simulink model "motorCC"  (R2017b)
settings: Solver=VariableStepAuto  StartTime=0.0  StopTime=5.0  RelTol=1e-3
settings Model: Creator=Sofia  LastModifiedBy=Sofia

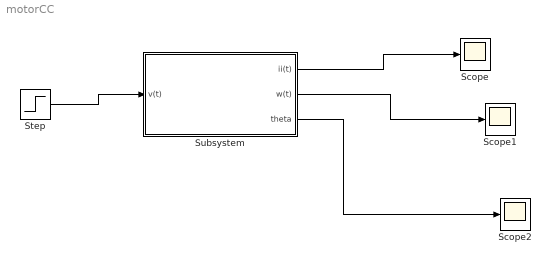
== system motorCC ==
  Scope : Scope
  Scope1 : Scope
  Scope2 : Scope
  Step : Step  After=5  SampleTime=0
  Subsystem : Subsystem
  wires:
  Step/1 -> Subsystem/1(v(t))
  Subsystem/1(ii(t)) -> Scope/1
  Subsystem/2(w(t)) -> Scope1/1
  Subsystem/3(theta) -> Scope2/1

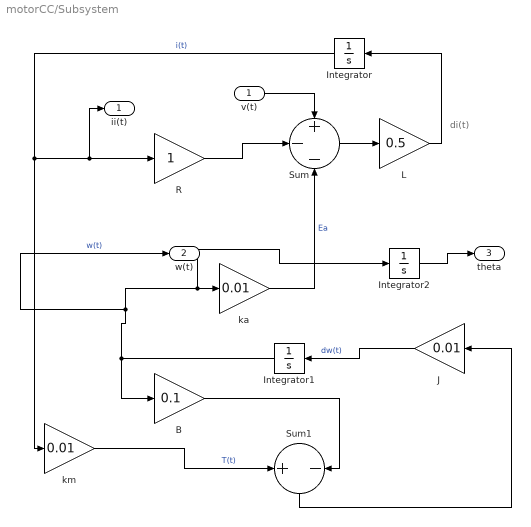
== system motorCC/Subsystem ==
  note: di(t)
  v(t) : Inport
  B : Gain  Gain=0.1
  Integrator : Integrator
  Integrator1 : Integrator
  Integrator2 : Integrator
  J : Gain  Gain=0.01
  L : Gain  Gain=0.5
  R : Gain
  Sum : Sum  Inputs=+--
  Sum1 : Sum  Inputs=+-
  ka : Gain  Gain=0.01
  km : Gain  Gain=0.01
  ii(t) : Outport
  w(t) : Outport  Port=2
  theta : Outport  Port=3
  wires:
  Integrator1/1 -> B/1, w(t)/1, Integrator2/1, ka/1  "w(t)"
  Integrator/1 -> km/1, ii(t)/1, R/1  "i(t)"
  Sum/1 -> L/1
  ka/1 -> Sum/3  "Ea"
  Integrator2/1 -> theta/1
  v(t)/1 -> Sum/1
  L/1 -> Integrator/1
  Sum1/1 -> J/1
  J/1 -> Integrator1/1  "dw(t)"
  km/1 -> Sum1/1  "T(t)"
  R/1 -> Sum/2
  B/1 -> Sum1/2
